simulink model "cartPendulum"  (R2019b)
settings: Solver=VariableStepAuto  StartTime=0.0  StopTime=100  RelTol=1e-3
values from neighbouring files (symbols this model uses):
  K = lqr(A, B, R, Q, N)    [generateResults.m]    (also in main.m)
undefined symbols (not defined in the file or in its folder): X0
libraries: simulink_extras x2
settings Model: Creator=emiel  LastModifiedBy=emiel

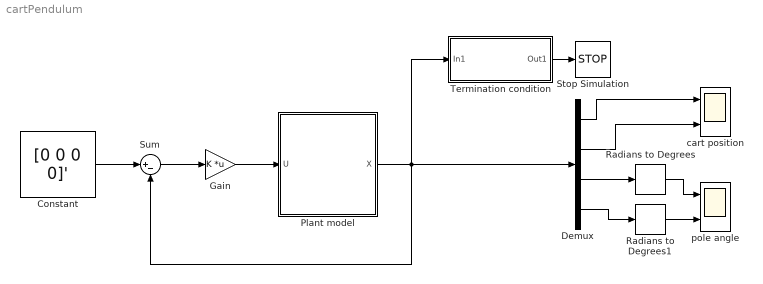
== system cartPendulum ==
  Constant : Constant  Value=[0 0 0 0]'
  Demux : Demux
  Gain : Gain  Gain=K  Multiplication=Matrix(K*u)
  Plant model : Subsystem
  Radians to Degrees : simulink_extras/Transformations/Radians to Degrees
  Radians to Degrees1 : simulink_extras/Transformations/Radians to Degrees
  Stop Simulation : Stop
  Sum : Sum  Inputs=|+-
  Termination condition : Subsystem
  cart position : Scope  NumInputPorts=2
  pole angle : Scope  NumInputPorts=2
  wires:
  Demux/1 -> cart position/1
  Demux/2 -> cart position/2
  Plant model/1(X) -> Sum/2, Demux/1, Termination condition/1(In1)
  Sum/1 -> Gain/1
  Gain/1 -> Plant model/1(U)
  Constant/1 -> Sum/1
  Termination condition/1(Out1) -> Stop Simulation/1
  Demux/3 -> Radians to Degrees/1
  Radians to Degrees/1 -> pole angle/1
  Demux/4 -> Radians to Degrees1/1
  Radians to Degrees1/1 -> pole angle/2

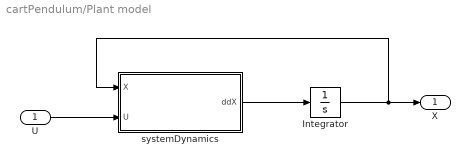
== system cartPendulum/Plant model ==
  U : Inport
  Integrator : Integrator  InitialCondition=X0
  systemDynamics : MATLAB Function  TreatAsAtomicUnit=on
  X : Outport
  wires:
  systemDynamics/1(ddX) -> Integrator/1
  U/1 -> systemDynamics/2(U)
  Integrator/1 -> systemDynamics/1(X), X/1

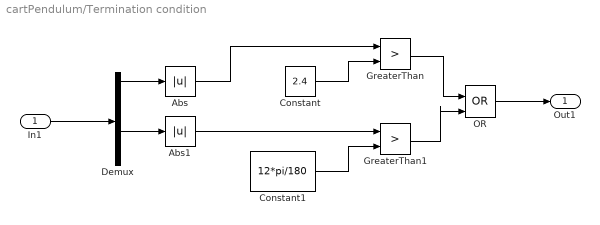
== system cartPendulum/Termination condition ==
  In1 : Inport
  Abs : Abs
  Abs1 : Abs
  Constant : Constant  Value=2.4
  Constant1 : Constant  Value=12*pi/180
  Demux : Demux
  GreaterThan : RelationalOperator  Operator=>  OutDataTypeStr=boolean  RndMeth=Simplest
  GreaterThan1 : RelationalOperator  Operator=>  OutDataTypeStr=boolean  RndMeth=Simplest
  OR : Logic  Operator=OR  IconShape=distinctive  AllPortsSameDT=off  OutDataTypeStr=boolean
  Out1 : Outport
  wires:
  In1/1 -> Demux/1
  GreaterThan/1 -> OR/1
  Demux/1 -> Abs/1
  GreaterThan1/1 -> OR/2
  OR/1 -> Out1/1
  Demux/3 -> Abs1/1
  Abs1/1 -> GreaterThan1/1
  Abs/1 -> GreaterThan/1
  Constant/1 -> GreaterThan/2
  Constant1/1 -> GreaterThan1/2

== matlab function cartPendulum/Plant model/systemDynamics ==
  data: X input size=4; ddX output size=4; U input; param parameter
function ddX = fcn(X, U, param)
% System Dynamics
%   State space representation of the car-pole system dynamics. X and dX
%   refer to the state vectors, and not to the position of the cart.
%   Param contains system parameters such as the cart and pole mass,
%   friction coefficients etc. 
%       X = state vector
%       X = [x, dx/dt, theta, dtheta/dt]'
        
    d2theta = (param.sys.g*sin(X(3)) ...
           + cos(X(3))*(-U - param.sys.m*param.sys.l*X(4)^2*sin(X(3)) + param.sys.muc*sign(X(2)))/(param.sys.m + param.sys.mc) ...
           - param.sys.mup*X(4)/param.sys.m/param.sys.l)/param.sys.l/(4/3 - (param.sys.m*cos(X(3))^2)/(param.sys.m + param.sys.mc));
       
    d2x = (U + param.sys.m*param.sys.l*(X(4)^2*sin(X(3)) - d2theta*cos(X(3))) - param.sys.muc*sign(X(2)))/(param.sys.m + param.sys.mc);
    
    ddX = [X(2) d2x X(4) d2theta]';
end
